simulink model "HybridFEMModel"  (Simulink 7.0)
settings: Solver=FixedStepDiscrete  SolverMode=SingleTasking  StartTime=0.0  StopTime=RunningTime  FixedStep=SampleRate  RelTol=1e-3
undefined symbols (not defined in the file): Alpham, DiscIntNeverNeededParam, Elements, gamma1, gamma2, sample, SampleRate
libraries: simulink x6
(part 2 of 4)

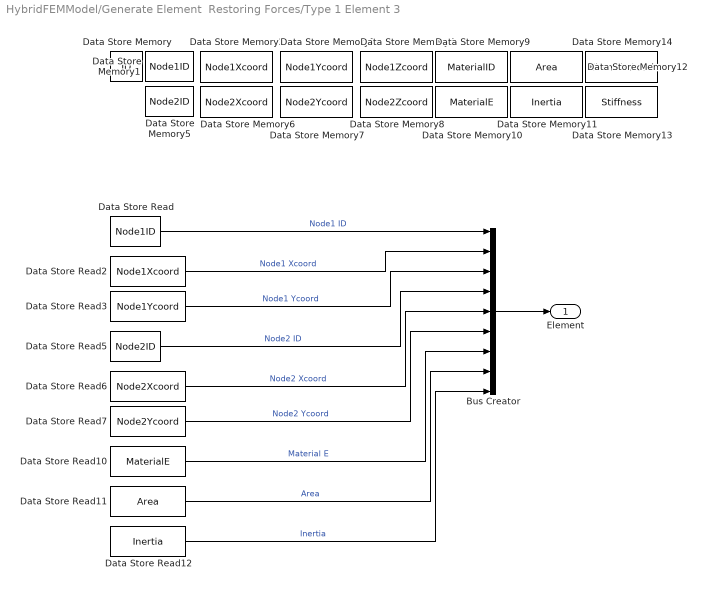
== system HybridFEMModel/Generate Element  Restoring Forces/Type 1 Element 3 ==
  Bus Creator : BusCreator  Inputs=9
  Data Store Memory : DataStoreMemory  DataStoreName=ID  InitialValue=Elements(id).ID  OutDataType=sfix(16)  OutScaling=2^0
  Data Store Memory1 : DataStoreMemory  DataStoreName=Node1ID  InitialValue=Elements(id).Nodes(1).ID  OutDataType=sfix(16)  OutScaling=2^0
  Data Store Memory10 : DataStoreMemory  DataStoreName=MaterialE  InitialValue=Elements(id).Material(1).E  OutDataType=sfix(16)  OutScaling=2^0
  Data Store Memory11 : DataStoreMemory  DataStoreName=Inertia  InitialValue=Elements(id).Inertia  OutDataType=sfix(16)  OutScaling=2^0
  Data Store Memory12 : DataStoreMemory  DataStoreName=Area  InitialValue=Elements(id).Area  OutDataType=sfix(16)  OutScaling=2^0
  Data Store Memory13 : DataStoreMemory  DataStoreName=Stiffness  InitialValue=Elements(id).Stiffness  OutDataType=sfix(16)  OutScaling=2^0
  Data Store Memory14 : DataStoreMemory  DataStoreName=ElemDistLoad  InitialValue=Elements(id).ElemDistLoad  OutDataType=sfix(16)  OutScaling=2^0
  Data Store Memory2 : DataStoreMemory  DataStoreName=Node1Xcoord  InitialValue=Elements(id).Nodes(1).Xcoord  OutDataType=sfix(16)  OutScaling=2^0
  Data Store Memory3 : DataStoreMemory  DataStoreName=Node1Ycoord  InitialValue=Elements(id).Nodes(1).Ycoord  OutDataType=sfix(16)  OutScaling=2^0
  Data Store Memory4 : DataStoreMemory  DataStoreName=Node1Zcoord  InitialValue=Elements(id).Nodes(1).Zcoord  OutDataType=sfix(16)  OutScaling=2^0
  Data Store Memory5 : DataStoreMemory  DataStoreName=Node2ID  InitialValue=Elements(id).Nodes(2).ID  OutDataType=sfix(16)  OutScaling=2^0
  Data Store Memory6 : DataStoreMemory  DataStoreName=Node2Xcoord  InitialValue=Elements(id).Nodes(2).Xcoord  OutDataType=sfix(16)  OutScaling=2^0
  Data Store Memory7 : DataStoreMemory  DataStoreName=Node2Ycoord  InitialValue=Elements(id).Nodes(2).Ycoord  OutDataType=sfix(16)  OutScaling=2^0
  Data Store Memory8 : DataStoreMemory  DataStoreName=Node2Zcoord  InitialValue=Elements(id).Nodes(2).Zcoord  OutDataType=sfix(16)  OutScaling=2^0
  Data Store Memory9 : DataStoreMemory  DataStoreName=MaterialID  InitialValue=Elements(id).Material(1).ID  OutDataType=sfix(16)  OutScaling=2^0
  Data Store Read : DataStoreRead  DataStoreName=Node1ID  SampleTime=-1
  Data Store Read10 : DataStoreRead  DataStoreName=MaterialE  SampleTime=-1
  Data Store Read11 : DataStoreRead  DataStoreName=Area  SampleTime=-1
  Data Store Read12 : DataStoreRead  DataStoreName=Inertia  SampleTime=-1
  Data Store Read2 : DataStoreRead  DataStoreName=Node1Xcoord  SampleTime=-1
  Data Store Read3 : DataStoreRead  DataStoreName=Node1Ycoord  SampleTime=-1
  Data Store Read5 : DataStoreRead  DataStoreName=Node2ID  SampleTime=-1
  Data Store Read6 : DataStoreRead  DataStoreName=Node2Xcoord  SampleTime=-1
  Data Store Read7 : DataStoreRead  DataStoreName=Node2Ycoord  SampleTime=-1
  Element : Outport  OutDataType=sfix(16)  OutScaling=2^0
  wires:
  Data Store Read12/1 -> Bus Creator/9  "Inertia"
  Data Store Read11/1 -> Bus Creator/8  "Area"
  Data Store Read10/1 -> Bus Creator/7  "Material E"
  Data Store Read7/1 -> Bus Creator/6  "Node2 Ycoord"
  Data Store Read6/1 -> Bus Creator/5  "Node2 Xcoord"
  Data Store Read5/1 -> Bus Creator/4  "Node2 ID"
  Data Store Read3/1 -> Bus Creator/3  "Node1 Ycoord"
  Data Store Read2/1 -> Bus Creator/2  "Node1 Xcoord"
  Data Store Read/1 -> Bus Creator/1  "Node1 ID"
  Bus Creator/1 -> Element/1

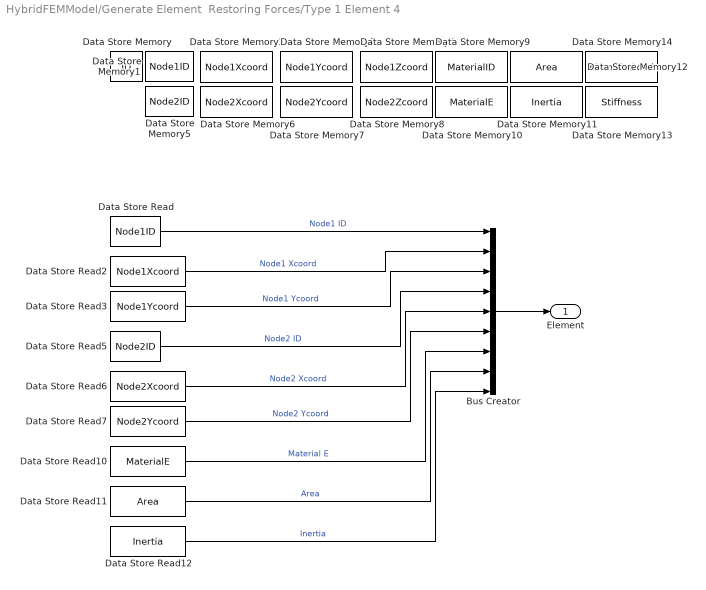
== system HybridFEMModel/Generate Element  Restoring Forces/Type 1 Element 4 ==
  Bus Creator : BusCreator  Inputs=9
  Data Store Memory : DataStoreMemory  DataStoreName=ID  InitialValue=Elements(id).ID  OutDataType=sfix(16)  OutScaling=2^0
  Data Store Memory1 : DataStoreMemory  DataStoreName=Node1ID  InitialValue=Elements(id).Nodes(1).ID  OutDataType=sfix(16)  OutScaling=2^0
  Data Store Memory10 : DataStoreMemory  DataStoreName=MaterialE  InitialValue=Elements(id).Material(1).E  OutDataType=sfix(16)  OutScaling=2^0
  Data Store Memory11 : DataStoreMemory  DataStoreName=Inertia  InitialValue=Elements(id).Inertia  OutDataType=sfix(16)  OutScaling=2^0
  Data Store Memory12 : DataStoreMemory  DataStoreName=Area  InitialValue=Elements(id).Area  OutDataType=sfix(16)  OutScaling=2^0
  Data Store Memory13 : DataStoreMemory  DataStoreName=Stiffness  InitialValue=Elements(id).Stiffness  OutDataType=sfix(16)  OutScaling=2^0
  Data Store Memory14 : DataStoreMemory  DataStoreName=ElemDistLoad  InitialValue=Elements(id).ElemDistLoad  OutDataType=sfix(16)  OutScaling=2^0
  Data Store Memory2 : DataStoreMemory  DataStoreName=Node1Xcoord  InitialValue=Elements(id).Nodes(1).Xcoord  OutDataType=sfix(16)  OutScaling=2^0
  Data Store Memory3 : DataStoreMemory  DataStoreName=Node1Ycoord  InitialValue=Elements(id).Nodes(1).Ycoord  OutDataType=sfix(16)  OutScaling=2^0
  Data Store Memory4 : DataStoreMemory  DataStoreName=Node1Zcoord  InitialValue=Elements(id).Nodes(1).Zcoord  OutDataType=sfix(16)  OutScaling=2^0
  Data Store Memory5 : DataStoreMemory  DataStoreName=Node2ID  InitialValue=Elements(id).Nodes(2).ID  OutDataType=sfix(16)  OutScaling=2^0
  Data Store Memory6 : DataStoreMemory  DataStoreName=Node2Xcoord  InitialValue=Elements(id).Nodes(2).Xcoord  OutDataType=sfix(16)  OutScaling=2^0
  Data Store Memory7 : DataStoreMemory  DataStoreName=Node2Ycoord  InitialValue=Elements(id).Nodes(2).Ycoord  OutDataType=sfix(16)  OutScaling=2^0
  Data Store Memory8 : DataStoreMemory  DataStoreName=Node2Zcoord  InitialValue=Elements(id).Nodes(2).Zcoord  OutDataType=sfix(16)  OutScaling=2^0
  Data Store Memory9 : DataStoreMemory  DataStoreName=MaterialID  InitialValue=Elements(id).Material(1).ID  OutDataType=sfix(16)  OutScaling=2^0
  Data Store Read : DataStoreRead  DataStoreName=Node1ID  SampleTime=-1
  Data Store Read10 : DataStoreRead  DataStoreName=MaterialE  SampleTime=-1
  Data Store Read11 : DataStoreRead  DataStoreName=Area  SampleTime=-1
  Data Store Read12 : DataStoreRead  DataStoreName=Inertia  SampleTime=-1
  Data Store Read2 : DataStoreRead  DataStoreName=Node1Xcoord  SampleTime=-1
  Data Store Read3 : DataStoreRead  DataStoreName=Node1Ycoord  SampleTime=-1
  Data Store Read5 : DataStoreRead  DataStoreName=Node2ID  SampleTime=-1
  Data Store Read6 : DataStoreRead  DataStoreName=Node2Xcoord  SampleTime=-1
  Data Store Read7 : DataStoreRead  DataStoreName=Node2Ycoord  SampleTime=-1
  Element : Outport  OutDataType=sfix(16)  OutScaling=2^0
  wires:
  Bus Creator/1 -> Element/1
  Data Store Read/1 -> Bus Creator/1  "Node1 ID"
  Data Store Read2/1 -> Bus Creator/2  "Node1 Xcoord"
  Data Store Read3/1 -> Bus Creator/3  "Node1 Ycoord"
  Data Store Read5/1 -> Bus Creator/4  "Node2 ID"
  Data Store Read6/1 -> Bus Creator/5  "Node2 Xcoord"
  Data Store Read7/1 -> Bus Creator/6  "Node2 Ycoord"
  Data Store Read10/1 -> Bus Creator/7  "Material E"
  Data Store Read11/1 -> Bus Creator/8  "Area"
  Data Store Read12/1 -> Bus Creator/9  "Inertia"

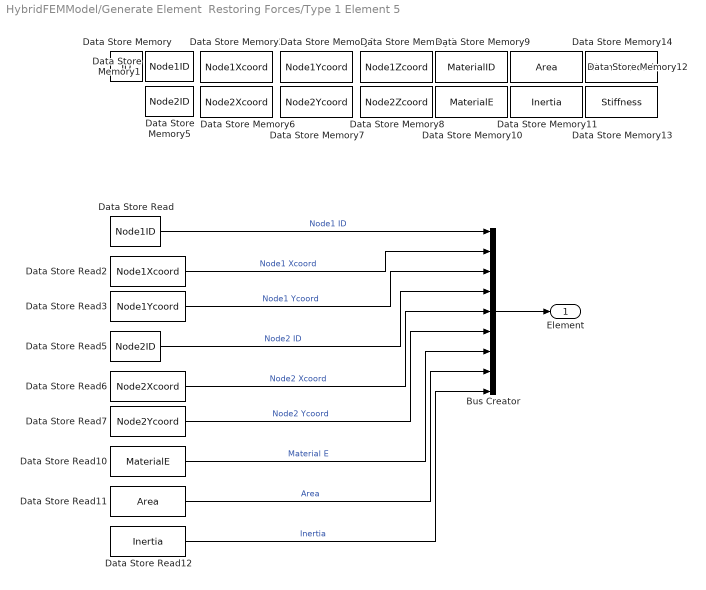
== system HybridFEMModel/Generate Element  Restoring Forces/Type 1 Element 5 ==
  Bus Creator : BusCreator  Inputs=9
  Data Store Memory : DataStoreMemory  DataStoreName=ID  InitialValue=Elements(id).ID  OutDataType=sfix(16)  OutScaling=2^0
  Data Store Memory1 : DataStoreMemory  DataStoreName=Node1ID  InitialValue=Elements(id).Nodes(1).ID  OutDataType=sfix(16)  OutScaling=2^0
  Data Store Memory10 : DataStoreMemory  DataStoreName=MaterialE  InitialValue=Elements(id).Material(1).E  OutDataType=sfix(16)  OutScaling=2^0
  Data Store Memory11 : DataStoreMemory  DataStoreName=Inertia  InitialValue=Elements(id).Inertia  OutDataType=sfix(16)  OutScaling=2^0
  Data Store Memory12 : DataStoreMemory  DataStoreName=Area  InitialValue=Elements(id).Area  OutDataType=sfix(16)  OutScaling=2^0
  Data Store Memory13 : DataStoreMemory  DataStoreName=Stiffness  InitialValue=Elements(id).Stiffness  OutDataType=sfix(16)  OutScaling=2^0
  Data Store Memory14 : DataStoreMemory  DataStoreName=ElemDistLoad  InitialValue=Elements(id).ElemDistLoad  OutDataType=sfix(16)  OutScaling=2^0
  Data Store Memory2 : DataStoreMemory  DataStoreName=Node1Xcoord  InitialValue=Elements(id).Nodes(1).Xcoord  OutDataType=sfix(16)  OutScaling=2^0
  Data Store Memory3 : DataStoreMemory  DataStoreName=Node1Ycoord  InitialValue=Elements(id).Nodes(1).Ycoord  OutDataType=sfix(16)  OutScaling=2^0
  Data Store Memory4 : DataStoreMemory  DataStoreName=Node1Zcoord  InitialValue=Elements(id).Nodes(1).Zcoord  OutDataType=sfix(16)  OutScaling=2^0
  Data Store Memory5 : DataStoreMemory  DataStoreName=Node2ID  InitialValue=Elements(id).Nodes(2).ID  OutDataType=sfix(16)  OutScaling=2^0
  Data Store Memory6 : DataStoreMemory  DataStoreName=Node2Xcoord  InitialValue=Elements(id).Nodes(2).Xcoord  OutDataType=sfix(16)  OutScaling=2^0
  Data Store Memory7 : DataStoreMemory  DataStoreName=Node2Ycoord  InitialValue=Elements(id).Nodes(2).Ycoord  OutDataType=sfix(16)  OutScaling=2^0
  Data Store Memory8 : DataStoreMemory  DataStoreName=Node2Zcoord  InitialValue=Elements(id).Nodes(2).Zcoord  OutDataType=sfix(16)  OutScaling=2^0
  Data Store Memory9 : DataStoreMemory  DataStoreName=MaterialID  InitialValue=Elements(id).Material(1).ID  OutDataType=sfix(16)  OutScaling=2^0
  Data Store Read : DataStoreRead  DataStoreName=Node1ID  SampleTime=-1
  Data Store Read10 : DataStoreRead  DataStoreName=MaterialE  SampleTime=-1
  Data Store Read11 : DataStoreRead  DataStoreName=Area  SampleTime=-1
  Data Store Read12 : DataStoreRead  DataStoreName=Inertia  SampleTime=-1
  Data Store Read2 : DataStoreRead  DataStoreName=Node1Xcoord  SampleTime=-1
  Data Store Read3 : DataStoreRead  DataStoreName=Node1Ycoord  SampleTime=-1
  Data Store Read5 : DataStoreRead  DataStoreName=Node2ID  SampleTime=-1
  Data Store Read6 : DataStoreRead  DataStoreName=Node2Xcoord  SampleTime=-1
  Data Store Read7 : DataStoreRead  DataStoreName=Node2Ycoord  SampleTime=-1
  Element : Outport  OutDataType=sfix(16)  OutScaling=2^0
  wires:
  Data Store Read12/1 -> Bus Creator/9  "Inertia"
  Data Store Read11/1 -> Bus Creator/8  "Area"
  Data Store Read10/1 -> Bus Creator/7  "Material E"
  Data Store Read7/1 -> Bus Creator/6  "Node2 Ycoord"
  Data Store Read6/1 -> Bus Creator/5  "Node2 Xcoord"
  Data Store Read5/1 -> Bus Creator/4  "Node2 ID"
  Data Store Read3/1 -> Bus Creator/3  "Node1 Ycoord"
  Data Store Read2/1 -> Bus Creator/2  "Node1 Xcoord"
  Data Store Read/1 -> Bus Creator/1  "Node1 ID"
  Bus Creator/1 -> Element/1

== system HybridFEMModel/Generate Element  Restoring Forces/Type 2 Element ==
  Bus Creator : BusCreator  Inputs=3
  Data Store Memory : DataStoreMemory  DataStoreName=ID  InitialValue=Elements(id).ID  OutDataType=sfix(16)  OutScaling=2^0
  Data Store Memory1 : DataStoreMemory  DataStoreName=Node1ID  InitialValue=Elements(id).Nodes(1).ID  OutDataType=sfix(16)  OutScaling=2^0
  Data Store Memory10 : DataStoreMemory  DataStoreName=MaterialE  InitialValue=Elements(id).Material(1).E  OutDataType=sfix(16)  OutScaling=2^0
  Data Store Memory11 : DataStoreMemory  DataStoreName=Inertia  InitialValue=Elements(id).Inertia  OutDataType=sfix(16)  OutScaling=2^0
  Data Store Memory12 : DataStoreMemory  DataStoreName=Area  InitialValue=Elements(id).Area  OutDataType=sfix(16)  OutScaling=2^0
  Data Store Memory13 : DataStoreMemory  DataStoreName=Stiffness  InitialValue=Elements(id).Stiffness  OutDataType=sfix(16)  OutScaling=2^0
  Data Store Memory14 : DataStoreMemory  DataStoreName=ElemDistLoad  InitialValue=Elements(id).ElemDistLoad  OutDataType=sfix(16)  OutScaling=2^0
  Data Store Memory2 : DataStoreMemory  DataStoreName=Node1Xcoord  InitialValue=Elements(id).Nodes(1).Xcoord  OutDataType=sfix(16)  OutScaling=2^0
  Data Store Memory3 : DataStoreMemory  DataStoreName=Node1Ycoord  InitialValue=Elements(id).Nodes(1).Ycoord  OutDataType=sfix(16)  OutScaling=2^0
  Data Store Memory4 : DataStoreMemory  DataStoreName=Node1Zcoord  InitialValue=Elements(id).Nodes(1).Zcoord  OutDataType=sfix(16)  OutScaling=2^0
  Data Store Memory5 : DataStoreMemory  DataStoreName=Node2ID  InitialValue=Elements(id).Nodes(2).ID  OutDataType=sfix(16)  OutScaling=2^0
  Data Store Memory6 : DataStoreMemory  DataStoreName=Node2Xcoord  InitialValue=Elements(id).Nodes(2).Xcoord  OutDataType=sfix(16)  OutScaling=2^0
  Data Store Memory7 : DataStoreMemory  DataStoreName=Node2Ycoord  InitialValue=Elements(id).Nodes(2).Ycoord  OutDataType=sfix(16)  OutScaling=2^0
  Data Store Memory8 : DataStoreMemory  DataStoreName=Node2Zcoord  InitialValue=Elements(id).Nodes(2).Zcoord  OutDataType=sfix(16)  OutScaling=2^0
  Data Store Memory9 : DataStoreMemory  DataStoreName=MaterialID  InitialValue=Elements(id).Material(1).ID  OutDataType=sfix(16)  OutScaling=2^0
  Data Store Read : DataStoreRead  DataStoreName=Node1ID  SampleTime=-1
  Data Store Read14 : DataStoreRead  DataStoreName=Stiffness  SampleTime=-1
  Data Store Read5 : DataStoreRead  DataStoreName=Node2ID  SampleTime=-1
  Element : Outport  OutDataType=sfix(16)  OutScaling=2^0
  wires:
  Data Store Read14/1 -> Bus Creator/3  "Stiffness"
  Data Store Read5/1 -> Bus Creator/2  "Node2 ID"
  Data Store Read/1 -> Bus Creator/1  "Node1 ID"
  Bus Creator/1 -> Element/1

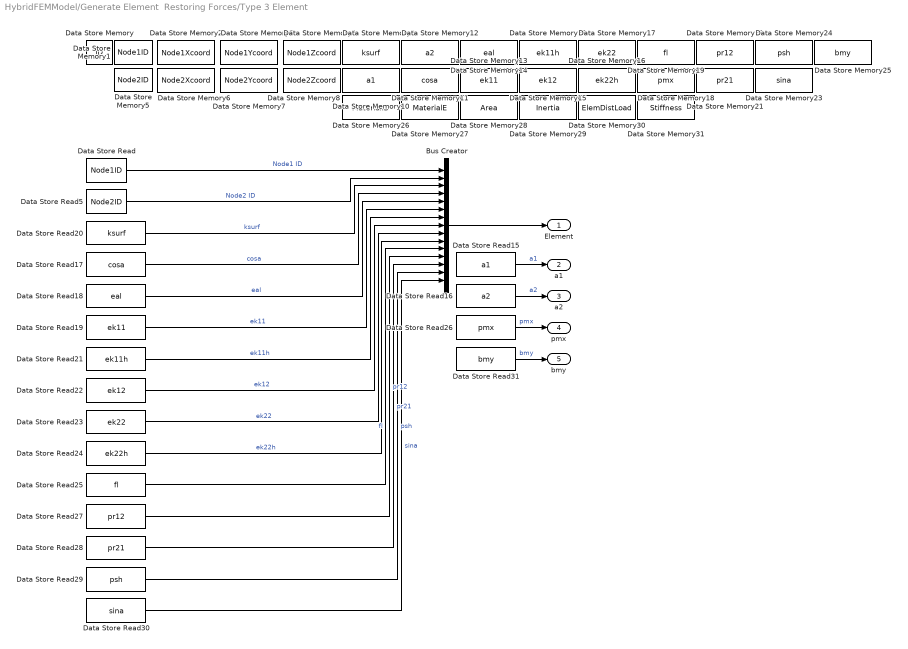
== system HybridFEMModel/Generate Element  Restoring Forces/Type 3 Element  ==
  Bus Creator : BusCreator  Inputs=15
  Data Store Memory : DataStoreMemory  DataStoreName=ID  InitialValue=Elements(id).ID  OutDataType=sfix(16)  OutScaling=2^0
  Data Store Memory1 : DataStoreMemory  DataStoreName=Node1ID  InitialValue=Elements(id).Nodes(1).ID  OutDataType=sfix(16)  OutScaling=2^0
  Data Store Memory10 : DataStoreMemory  DataStoreName=a1  InitialValue=Elements(id).a1  OutDataType=sfix(16)  OutScaling=2^0
  Data Store Memory11 : DataStoreMemory  DataStoreName=cosa  InitialValue=Elements(id).cosa  OutDataType=sfix(16)  OutScaling=2^0
  Data Store Memory12 : DataStoreMemory  DataStoreName=a2  InitialValue=Elements(id).a2  OutDataType=sfix(16)  OutScaling=2^0
  Data Store Memory13 : DataStoreMemory  DataStoreName=ek11  InitialValue=Elements(id).ek11  OutDataType=sfix(16)  OutScaling=2^0
  Data Store Memory14 : DataStoreMemory  DataStoreName=eal  InitialValue=Elements(id).eal  OutDataType=sfix(16)  OutScaling=2^0
  Data Store Memory15 : DataStoreMemory  DataStoreName=ek12  InitialValue=Elements(id).ek12  OutDataType=sfix(16)  OutScaling=2^0
  Data Store Memory16 : DataStoreMemory  DataStoreName=ek22h  InitialValue=Elements(id).ek22h  OutDataType=sfix(16)  OutScaling=2^0
  Data Store Memory17 : DataStoreMemory  DataStoreName=ek22  InitialValue=Elements(id).ek22  OutDataType=sfix(16)  OutScaling=2^0
  Data Store Memory18 : DataStoreMemory  DataStoreName=pmx  InitialValue=Elements(id).pmx  OutDataType=sfix(16)  OutScaling=2^0
  Data Store Memory19 : DataStoreMemory  DataStoreName=fl  InitialValue=Elements(id).fl  OutDataType=sfix(16)  OutScaling=2^0
  Data Store Memory2 : DataStoreMemory  DataStoreName=Node1Xcoord  InitialValue=Elements(id).Nodes(1).Xcoord  OutDataType=sfix(16)  OutScaling=2^0
  Data Store Memory20 : DataStoreMemory  DataStoreName=ek11h  InitialValue=Elements(id).ek11h  OutDataType=sfix(16)  OutScaling=2^0
  Data Store Memory21 : DataStoreMemory  DataStoreName=pr21  InitialValue=Elements(id).pr21  OutDataType=sfix(16)  OutScaling=2^0
  Data Store Memory22 : DataStoreMemory  DataStoreName=pr12  InitialValue=Elements(id).pr12  OutDataType=sfix(16)  OutScaling=2^0
  Data Store Memory23 : DataStoreMemory  DataStoreName=sina  InitialValue=Elements(id).sina  OutDataType=sfix(16)  OutScaling=2^0
  Data Store Memory24 : DataStoreMemory  DataStoreName=psh  InitialValue=Elements(id).psh  OutDataType=sfix(16)  OutScaling=2^0
  Data Store Memory25 : DataStoreMemory  DataStoreName=bmy  InitialValue=Elements(id).bmy  OutDataType=sfix(16)  OutScaling=2^0
  Data Store Memory26 : DataStoreMemory  DataStoreName=MaterialID  InitialValue=Elements(id).Material.ID  OutDataType=sfix(16)  OutScaling=2^0
  Data Store Memory27 : DataStoreMemory  DataStoreName=MaterialE  InitialValue=Elements(id).Material.E  OutDataType=sfix(16)  OutScaling=2^0
  Data Store Memory28 : DataStoreMemory  DataStoreName=Area  InitialValue=Elements(id).Area  OutDataType=sfix(16)  OutScaling=2^0
  Data Store Memory29 : DataStoreMemory  DataStoreName=Inertia  InitialValue=Elements(id).Inertia  OutDataType=sfix(16)  OutScaling=2^0
  Data Store Memory3 : DataStoreMemory  DataStoreName=Node1Ycoord  InitialValue=Elements(id).Nodes(1).Ycoord  OutDataType=sfix(16)  OutScaling=2^0
  Data Store Memory30 : DataStoreMemory  DataStoreName=ElemDistLoad  InitialValue=Elements(id).ElemDistLoad  OutDataType=sfix(16)  OutScaling=2^0
  Data Store Memory31 : DataStoreMemory  DataStoreName=Stiffness  InitialValue=Elements(id).Stiffness  OutDataType=sfix(16)  OutScaling=2^0
  Data Store Memory4 : DataStoreMemory  DataStoreName=Node1Zcoord  InitialValue=Elements(id).Nodes(1).Zcoord  OutDataType=sfix(16)  OutScaling=2^0
  Data Store Memory5 : DataStoreMemory  DataStoreName=Node2ID  InitialValue=Elements(id).Nodes(2).ID  OutDataType=sfix(16)  OutScaling=2^0
  Data Store Memory6 : DataStoreMemory  DataStoreName=Node2Xcoord  InitialValue=Elements(id).Nodes(2).Xcoord  OutDataType=sfix(16)  OutScaling=2^0
  Data Store Memory7 : DataStoreMemory  DataStoreName=Node2Ycoord  InitialValue=Elements(id).Nodes(2).Ycoord  OutDataType=sfix(16)  OutScaling=2^0
  Data Store Memory8 : DataStoreMemory  DataStoreName=Node2Zcoord  InitialValue=Elements(id).Nodes(2).Zcoord  OutDataType=sfix(16)  OutScaling=2^0
  Data Store Memory9 : DataStoreMemory  DataStoreName=ksurf  InitialValue=Elements(id).ksurf  OutDataType=sfix(16)  OutScaling=2^0
  Data Store Read : DataStoreRead  DataStoreName=Node1ID  SampleTime=-1
  Data Store Read15 : DataStoreRead  DataStoreName=a1  SampleTime=-1
  Data Store Read16 : DataStoreRead  DataStoreName=a2  SampleTime=-1
  Data Store Read17 : DataStoreRead  DataStoreName=cosa  SampleTime=-1
  Data Store Read18 : DataStoreRead  DataStoreName=eal  SampleTime=-1
  Data Store Read19 : DataStoreRead  DataStoreName=ek11  SampleTime=-1
  Data Store Read20 : DataStoreRead  DataStoreName=ksurf  SampleTime=-1
  Data Store Read21 : DataStoreRead  DataStoreName=ek11h  SampleTime=-1
  Data Store Read22 : DataStoreRead  DataStoreName=ek12  SampleTime=-1
  Data Store Read23 : DataStoreRead  DataStoreName=ek22  SampleTime=-1
  Data Store Read24 : DataStoreRead  DataStoreName=ek22h  SampleTime=-1
  Data Store Read25 : DataStoreRead  DataStoreName=fl  SampleTime=-1
  Data Store Read26 : DataStoreRead  DataStoreName=pmx  SampleTime=-1
  Data Store Read27 : DataStoreRead  DataStoreName=pr12  SampleTime=-1
  Data Store Read28 : DataStoreRead  DataStoreName=pr21  SampleTime=-1
  Data Store Read29 : DataStoreRead  DataStoreName=psh  SampleTime=-1
  Data Store Read30 : DataStoreRead  DataStoreName=sina  SampleTime=-1
  Data Store Read31 : DataStoreRead  DataStoreName=bmy  SampleTime=-1
  Data Store Read5 : DataStoreRead  DataStoreName=Node2ID  SampleTime=-1
  Element : Outport  OutDataType=sfix(16)  OutScaling=2^0
  a1 : Outport  Port=2  OutDataType=sfix(16)  OutScaling=2^0
  a2 : Outport  Port=3  OutDataType=sfix(16)  OutScaling=2^0
  pmx : Outport  Port=4  OutDataType=sfix(16)  OutScaling=2^0
  bmy : Outport  Port=5  OutDataType=sfix(16)  OutScaling=2^0
  wires:
  Bus Creator/1 -> Element/1
  Data Store Read/1 -> Bus Creator/1  "Node1 ID"
  Data Store Read5/1 -> Bus Creator/2  "Node2 ID"
  Data Store Read20/1 -> Bus Creator/3  "ksurf"
  Data Store Read17/1 -> Bus Creator/4  "cosa"
  Data Store Read18/1 -> Bus Creator/5  "eal"
  Data Store Read19/1 -> Bus Creator/6  "ek11"
  Data Store Read21/1 -> Bus Creator/7  "ek11h"
  Data Store Read22/1 -> Bus Creator/8  "ek12"
  Data Store Read23/1 -> Bus Creator/9  "ek22"
  Data Store Read24/1 -> Bus Creator/10  "ek22h"
  Data Store Read25/1 -> Bus Creator/11  "fl"
  Data Store Read27/1 -> Bus Creator/12  "pr12"
  Data Store Read28/1 -> Bus Creator/13  "pr21"
  Data Store Read29/1 -> Bus Creator/14  "psh"
  Data Store Read30/1 -> Bus Creator/15  "sina"
  Data Store Read15/1 -> a1/1  "a1"
  Data Store Read16/1 -> a2/1  "a2"
  Data Store Read26/1 -> pmx/1  "pmx"
  Data Store Read31/1 -> bmy/1  "bmy"

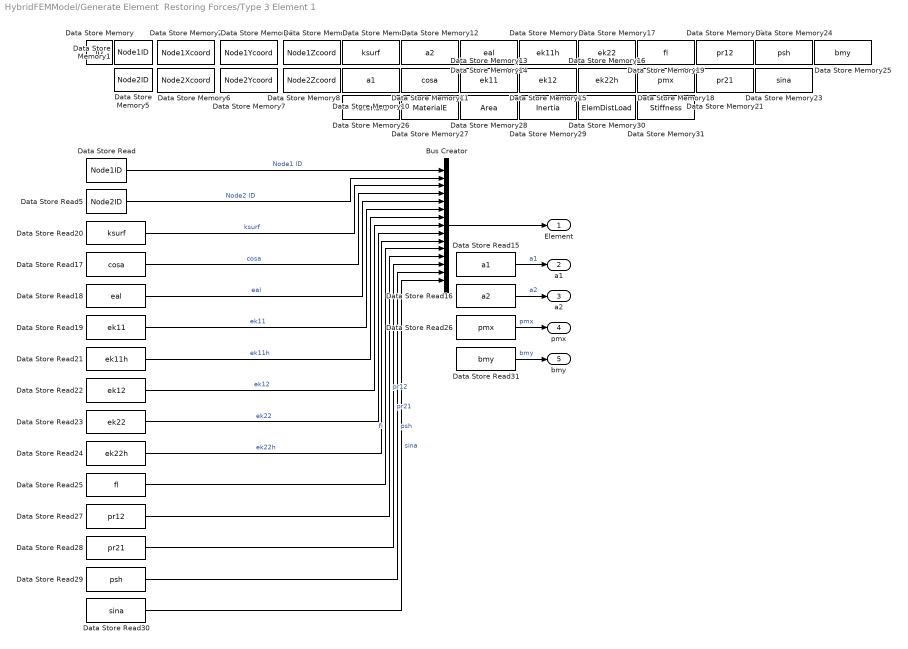
== system HybridFEMModel/Generate Element  Restoring Forces/Type 3 Element 1 ==
  Bus Creator : BusCreator  Inputs=15
  Data Store Memory : DataStoreMemory  DataStoreName=ID  InitialValue=Elements(id).ID  OutDataType=sfix(16)  OutScaling=2^0
  Data Store Memory1 : DataStoreMemory  DataStoreName=Node1ID  InitialValue=Elements(id).Nodes(1).ID  OutDataType=sfix(16)  OutScaling=2^0
  Data Store Memory10 : DataStoreMemory  DataStoreName=a1  InitialValue=Elements(id).a1  OutDataType=sfix(16)  OutScaling=2^0
  Data Store Memory11 : DataStoreMemory  DataStoreName=cosa  InitialValue=Elements(id).cosa  OutDataType=sfix(16)  OutScaling=2^0
  Data Store Memory12 : DataStoreMemory  DataStoreName=a2  InitialValue=Elements(id).a2  OutDataType=sfix(16)  OutScaling=2^0
  Data Store Memory13 : DataStoreMemory  DataStoreName=ek11  InitialValue=Elements(id).ek11  OutDataType=sfix(16)  OutScaling=2^0
  Data Store Memory14 : DataStoreMemory  DataStoreName=eal  InitialValue=Elements(id).eal  OutDataType=sfix(16)  OutScaling=2^0
  Data Store Memory15 : DataStoreMemory  DataStoreName=ek12  InitialValue=Elements(id).ek12  OutDataType=sfix(16)  OutScaling=2^0
  Data Store Memory16 : DataStoreMemory  DataStoreName=ek22h  InitialValue=Elements(id).ek22h  OutDataType=sfix(16)  OutScaling=2^0
  Data Store Memory17 : DataStoreMemory  DataStoreName=ek22  InitialValue=Elements(id).ek22  OutDataType=sfix(16)  OutScaling=2^0
  Data Store Memory18 : DataStoreMemory  DataStoreName=pmx  InitialValue=Elements(id).pmx  OutDataType=sfix(16)  OutScaling=2^0
  Data Store Memory19 : DataStoreMemory  DataStoreName=fl  InitialValue=Elements(id).fl  OutDataType=sfix(16)  OutScaling=2^0
  Data Store Memory2 : DataStoreMemory  DataStoreName=Node1Xcoord  InitialValue=Elements(id).Nodes(1).Xcoord  OutDataType=sfix(16)  OutScaling=2^0
  Data Store Memory20 : DataStoreMemory  DataStoreName=ek11h  InitialValue=Elements(id).ek11h  OutDataType=sfix(16)  OutScaling=2^0
  Data Store Memory21 : DataStoreMemory  DataStoreName=pr21  InitialValue=Elements(id).pr21  OutDataType=sfix(16)  OutScaling=2^0
  Data Store Memory22 : DataStoreMemory  DataStoreName=pr12  InitialValue=Elements(id).pr12  OutDataType=sfix(16)  OutScaling=2^0
  Data Store Memory23 : DataStoreMemory  DataStoreName=sina  InitialValue=Elements(id).sina  OutDataType=sfix(16)  OutScaling=2^0
  Data Store Memory24 : DataStoreMemory  DataStoreName=psh  InitialValue=Elements(id).psh  OutDataType=sfix(16)  OutScaling=2^0
  Data Store Memory25 : DataStoreMemory  DataStoreName=bmy  InitialValue=Elements(id).bmy  OutDataType=sfix(16)  OutScaling=2^0
  Data Store Memory26 : DataStoreMemory  DataStoreName=MaterialID  InitialValue=Elements(id).Material.ID  OutDataType=sfix(16)  OutScaling=2^0
  Data Store Memory27 : DataStoreMemory  DataStoreName=MaterialE  InitialValue=Elements(id).Material.E  OutDataType=sfix(16)  OutScaling=2^0
  Data Store Memory28 : DataStoreMemory  DataStoreName=Area  InitialValue=Elements(id).Area  OutDataType=sfix(16)  OutScaling=2^0
  Data Store Memory29 : DataStoreMemory  DataStoreName=Inertia  InitialValue=Elements(id).Inertia  OutDataType=sfix(16)  OutScaling=2^0
  Data Store Memory3 : DataStoreMemory  DataStoreName=Node1Ycoord  InitialValue=Elements(id).Nodes(1).Ycoord  OutDataType=sfix(16)  OutScaling=2^0
  Data Store Memory30 : DataStoreMemory  DataStoreName=ElemDistLoad  InitialValue=Elements(id).ElemDistLoad  OutDataType=sfix(16)  OutScaling=2^0
  Data Store Memory31 : DataStoreMemory  DataStoreName=Stiffness  InitialValue=Elements(id).Stiffness  OutDataType=sfix(16)  OutScaling=2^0
  Data Store Memory4 : DataStoreMemory  DataStoreName=Node1Zcoord  InitialValue=Elements(id).Nodes(1).Zcoord  OutDataType=sfix(16)  OutScaling=2^0
  Data Store Memory5 : DataStoreMemory  DataStoreName=Node2ID  InitialValue=Elements(id).Nodes(2).ID  OutDataType=sfix(16)  OutScaling=2^0
  Data Store Memory6 : DataStoreMemory  DataStoreName=Node2Xcoord  InitialValue=Elements(id).Nodes(2).Xcoord  OutDataType=sfix(16)  OutScaling=2^0
  Data Store Memory7 : DataStoreMemory  DataStoreName=Node2Ycoord  InitialValue=Elements(id).Nodes(2).Ycoord  OutDataType=sfix(16)  OutScaling=2^0
  Data Store Memory8 : DataStoreMemory  DataStoreName=Node2Zcoord  InitialValue=Elements(id).Nodes(2).Zcoord  OutDataType=sfix(16)  OutScaling=2^0
  Data Store Memory9 : DataStoreMemory  DataStoreName=ksurf  InitialValue=Elements(id).ksurf  OutDataType=sfix(16)  OutScaling=2^0
  Data Store Read : DataStoreRead  DataStoreName=Node1ID  SampleTime=-1
  Data Store Read15 : DataStoreRead  DataStoreName=a1  SampleTime=-1
  Data Store Read16 : DataStoreRead  DataStoreName=a2  SampleTime=-1
  Data Store Read17 : DataStoreRead  DataStoreName=cosa  SampleTime=-1
  Data Store Read18 : DataStoreRead  DataStoreName=eal  SampleTime=-1
  Data Store Read19 : DataStoreRead  DataStoreName=ek11  SampleTime=-1
  Data Store Read20 : DataStoreRead  DataStoreName=ksurf  SampleTime=-1
  Data Store Read21 : DataStoreRead  DataStoreName=ek11h  SampleTime=-1
  Data Store Read22 : DataStoreRead  DataStoreName=ek12  SampleTime=-1
  Data Store Read23 : DataStoreRead  DataStoreName=ek22  SampleTime=-1
  Data Store Read24 : DataStoreRead  DataStoreName=ek22h  SampleTime=-1
  Data Store Read25 : DataStoreRead  DataStoreName=fl  SampleTime=-1
  Data Store Read26 : DataStoreRead  DataStoreName=pmx  SampleTime=-1
  Data Store Read27 : DataStoreRead  DataStoreName=pr12  SampleTime=-1
  Data Store Read28 : DataStoreRead  DataStoreName=pr21  SampleTime=-1
  Data Store Read29 : DataStoreRead  DataStoreName=psh  SampleTime=-1
  Data Store Read30 : DataStoreRead  DataStoreName=sina  SampleTime=-1
  Data Store Read31 : DataStoreRead  DataStoreName=bmy  SampleTime=-1
  Data Store Read5 : DataStoreRead  DataStoreName=Node2ID  SampleTime=-1
  Element : Outport  OutDataType=sfix(16)  OutScaling=2^0
  a1 : Outport  Port=2  OutDataType=sfix(16)  OutScaling=2^0
  a2 : Outport  Port=3  OutDataType=sfix(16)  OutScaling=2^0
  pmx : Outport  Port=4  OutDataType=sfix(16)  OutScaling=2^0
  bmy : Outport  Port=5  OutDataType=sfix(16)  OutScaling=2^0
  wires:
  Data Store Read31/1 -> bmy/1  "bmy"
  Data Store Read26/1 -> pmx/1  "pmx"
  Data Store Read16/1 -> a2/1  "a2"
  Data Store Read15/1 -> a1/1  "a1"
  Data Store Read30/1 -> Bus Creator/15  "sina"
  Data Store Read29/1 -> Bus Creator/14  "psh"
  Data Store Read28/1 -> Bus Creator/13  "pr21"
  Data Store Read27/1 -> Bus Creator/12  "pr12"
  Data Store Read25/1 -> Bus Creator/11  "fl"
  Data Store Read24/1 -> Bus Creator/10  "ek22h"
  Data Store Read23/1 -> Bus Creator/9  "ek22"
  Data Store Read22/1 -> Bus Creator/8  "ek12"
  Data Store Read21/1 -> Bus Creator/7  "ek11h"
  Data Store Read19/1 -> Bus Creator/6  "ek11"
  Data Store Read18/1 -> Bus Creator/5  "eal"
  Data Store Read17/1 -> Bus Creator/4  "cosa"
  Data Store Read20/1 -> Bus Creator/3  "ksurf"
  Data Store Read5/1 -> Bus Creator/2  "Node2 ID"
  Data Store Read/1 -> Bus Creator/1  "Node1 ID"
  Bus Creator/1 -> Element/1

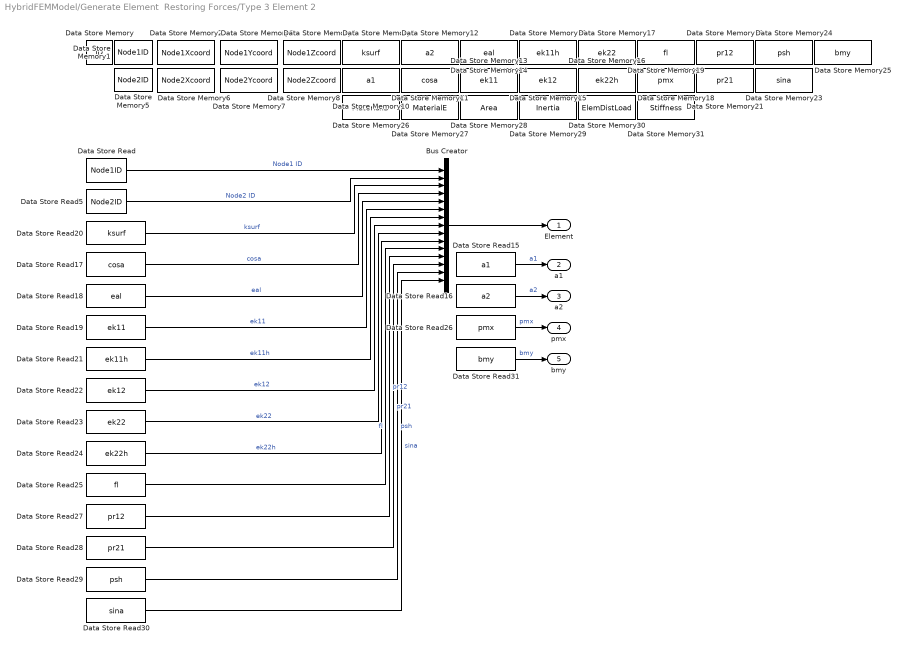
== system HybridFEMModel/Generate Element  Restoring Forces/Type 3 Element 2 ==
  Bus Creator : BusCreator  Inputs=15
  Data Store Memory : DataStoreMemory  DataStoreName=ID  InitialValue=Elements(id).ID  OutDataType=sfix(16)  OutScaling=2^0
  Data Store Memory1 : DataStoreMemory  DataStoreName=Node1ID  InitialValue=Elements(id).Nodes(1).ID  OutDataType=sfix(16)  OutScaling=2^0
  Data Store Memory10 : DataStoreMemory  DataStoreName=a1  InitialValue=Elements(id).a1  OutDataType=sfix(16)  OutScaling=2^0
  Data Store Memory11 : DataStoreMemory  DataStoreName=cosa  InitialValue=Elements(id).cosa  OutDataType=sfix(16)  OutScaling=2^0
  Data Store Memory12 : DataStoreMemory  DataStoreName=a2  InitialValue=Elements(id).a2  OutDataType=sfix(16)  OutScaling=2^0
  Data Store Memory13 : DataStoreMemory  DataStoreName=ek11  InitialValue=Elements(id).ek11  OutDataType=sfix(16)  OutScaling=2^0
  Data Store Memory14 : DataStoreMemory  DataStoreName=eal  InitialValue=Elements(id).eal  OutDataType=sfix(16)  OutScaling=2^0
  Data Store Memory15 : DataStoreMemory  DataStoreName=ek12  InitialValue=Elements(id).ek12  OutDataType=sfix(16)  OutScaling=2^0
  Data Store Memory16 : DataStoreMemory  DataStoreName=ek22h  InitialValue=Elements(id).ek22h  OutDataType=sfix(16)  OutScaling=2^0
  Data Store Memory17 : DataStoreMemory  DataStoreName=ek22  InitialValue=Elements(id).ek22  OutDataType=sfix(16)  OutScaling=2^0
  Data Store Memory18 : DataStoreMemory  DataStoreName=pmx  InitialValue=Elements(id).pmx  OutDataType=sfix(16)  OutScaling=2^0
  Data Store Memory19 : DataStoreMemory  DataStoreName=fl  InitialValue=Elements(id).fl  OutDataType=sfix(16)  OutScaling=2^0
  Data Store Memory2 : DataStoreMemory  DataStoreName=Node1Xcoord  InitialValue=Elements(id).Nodes(1).Xcoord  OutDataType=sfix(16)  OutScaling=2^0
  Data Store Memory20 : DataStoreMemory  DataStoreName=ek11h  InitialValue=Elements(id).ek11h  OutDataType=sfix(16)  OutScaling=2^0
  Data Store Memory21 : DataStoreMemory  DataStoreName=pr21  InitialValue=Elements(id).pr21  OutDataType=sfix(16)  OutScaling=2^0
  Data Store Memory22 : DataStoreMemory  DataStoreName=pr12  InitialValue=Elements(id).pr12  OutDataType=sfix(16)  OutScaling=2^0
  Data Store Memory23 : DataStoreMemory  DataStoreName=sina  InitialValue=Elements(id).sina  OutDataType=sfix(16)  OutScaling=2^0
  Data Store Memory24 : DataStoreMemory  DataStoreName=psh  InitialValue=Elements(id).psh  OutDataType=sfix(16)  OutScaling=2^0
  Data Store Memory25 : DataStoreMemory  DataStoreName=bmy  InitialValue=Elements(id).bmy  OutDataType=sfix(16)  OutScaling=2^0
  Data Store Memory26 : DataStoreMemory  DataStoreName=MaterialID  InitialValue=Elements(id).Material.ID  OutDataType=sfix(16)  OutScaling=2^0
  Data Store Memory27 : DataStoreMemory  DataStoreName=MaterialE  InitialValue=Elements(id).Material.E  OutDataType=sfix(16)  OutScaling=2^0
  Data Store Memory28 : DataStoreMemory  DataStoreName=Area  InitialValue=Elements(id).Area  OutDataType=sfix(16)  OutScaling=2^0
  Data Store Memory29 : DataStoreMemory  DataStoreName=Inertia  InitialValue=Elements(id).Inertia  OutDataType=sfix(16)  OutScaling=2^0
  Data Store Memory3 : DataStoreMemory  DataStoreName=Node1Ycoord  InitialValue=Elements(id).Nodes(1).Ycoord  OutDataType=sfix(16)  OutScaling=2^0
  Data Store Memory30 : DataStoreMemory  DataStoreName=ElemDistLoad  InitialValue=Elements(id).ElemDistLoad  OutDataType=sfix(16)  OutScaling=2^0
  Data Store Memory31 : DataStoreMemory  DataStoreName=Stiffness  InitialValue=Elements(id).Stiffness  OutDataType=sfix(16)  OutScaling=2^0
  Data Store Memory4 : DataStoreMemory  DataStoreName=Node1Zcoord  InitialValue=Elements(id).Nodes(1).Zcoord  OutDataType=sfix(16)  OutScaling=2^0
  Data Store Memory5 : DataStoreMemory  DataStoreName=Node2ID  InitialValue=Elements(id).Nodes(2).ID  OutDataType=sfix(16)  OutScaling=2^0
  Data Store Memory6 : DataStoreMemory  DataStoreName=Node2Xcoord  InitialValue=Elements(id).Nodes(2).Xcoord  OutDataType=sfix(16)  OutScaling=2^0
  Data Store Memory7 : DataStoreMemory  DataStoreName=Node2Ycoord  InitialValue=Elements(id).Nodes(2).Ycoord  OutDataType=sfix(16)  OutScaling=2^0
  Data Store Memory8 : DataStoreMemory  DataStoreName=Node2Zcoord  InitialValue=Elements(id).Nodes(2).Zcoord  OutDataType=sfix(16)  OutScaling=2^0
  Data Store Memory9 : DataStoreMemory  DataStoreName=ksurf  InitialValue=Elements(id).ksurf  OutDataType=sfix(16)  OutScaling=2^0
  Data Store Read : DataStoreRead  DataStoreName=Node1ID  SampleTime=-1
  Data Store Read15 : DataStoreRead  DataStoreName=a1  SampleTime=-1
  Data Store Read16 : DataStoreRead  DataStoreName=a2  SampleTime=-1
  Data Store Read17 : DataStoreRead  DataStoreName=cosa  SampleTime=-1
  Data Store Read18 : DataStoreRead  DataStoreName=eal  SampleTime=-1
  Data Store Read19 : DataStoreRead  DataStoreName=ek11  SampleTime=-1
  Data Store Read20 : DataStoreRead  DataStoreName=ksurf  SampleTime=-1
  Data Store Read21 : DataStoreRead  DataStoreName=ek11h  SampleTime=-1
  Data Store Read22 : DataStoreRead  DataStoreName=ek12  SampleTime=-1
  Data Store Read23 : DataStoreRead  DataStoreName=ek22  SampleTime=-1
  Data Store Read24 : DataStoreRead  DataStoreName=ek22h  SampleTime=-1
  Data Store Read25 : DataStoreRead  DataStoreName=fl  SampleTime=-1
  Data Store Read26 : DataStoreRead  DataStoreName=pmx  SampleTime=-1
  Data Store Read27 : DataStoreRead  DataStoreName=pr12  SampleTime=-1
  Data Store Read28 : DataStoreRead  DataStoreName=pr21  SampleTime=-1
  Data Store Read29 : DataStoreRead  DataStoreName=psh  SampleTime=-1
  Data Store Read30 : DataStoreRead  DataStoreName=sina  SampleTime=-1
  Data Store Read31 : DataStoreRead  DataStoreName=bmy  SampleTime=-1
  Data Store Read5 : DataStoreRead  DataStoreName=Node2ID  SampleTime=-1
  Element : Outport  OutDataType=sfix(16)  OutScaling=2^0
  a1 : Outport  Port=2  OutDataType=sfix(16)  OutScaling=2^0
  a2 : Outport  Port=3  OutDataType=sfix(16)  OutScaling=2^0
  pmx : Outport  Port=4  OutDataType=sfix(16)  OutScaling=2^0
  bmy : Outport  Port=5  OutDataType=sfix(16)  OutScaling=2^0
  wires:
  Bus Creator/1 -> Element/1
  Data Store Read/1 -> Bus Creator/1  "Node1 ID"
  Data Store Read5/1 -> Bus Creator/2  "Node2 ID"
  Data Store Read20/1 -> Bus Creator/3  "ksurf"
  Data Store Read17/1 -> Bus Creator/4  "cosa"
  Data Store Read18/1 -> Bus Creator/5  "eal"
  Data Store Read19/1 -> Bus Creator/6  "ek11"
  Data Store Read21/1 -> Bus Creator/7  "ek11h"
  Data Store Read22/1 -> Bus Creator/8  "ek12"
  Data Store Read23/1 -> Bus Creator/9  "ek22"
  Data Store Read24/1 -> Bus Creator/10  "ek22h"
  Data Store Read25/1 -> Bus Creator/11  "fl"
  Data Store Read27/1 -> Bus Creator/12  "pr12"
  Data Store Read28/1 -> Bus Creator/13  "pr21"
  Data Store Read29/1 -> Bus Creator/14  "psh"
  Data Store Read30/1 -> Bus Creator/15  "sina"
  Data Store Read15/1 -> a1/1  "a1"
  Data Store Read16/1 -> a2/1  "a2"
  Data Store Read26/1 -> pmx/1  "pmx"
  Data Store Read31/1 -> bmy/1  "bmy"

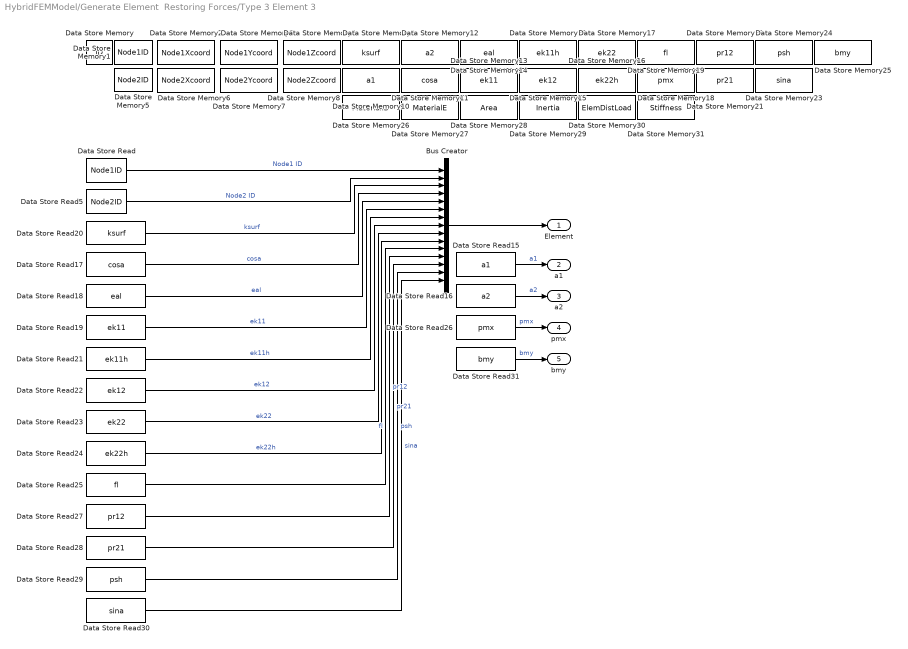
== system HybridFEMModel/Generate Element  Restoring Forces/Type 3 Element 3 ==
  Bus Creator : BusCreator  Inputs=15
  Data Store Memory : DataStoreMemory  DataStoreName=ID  InitialValue=Elements(id).ID  OutDataType=sfix(16)  OutScaling=2^0
  Data Store Memory1 : DataStoreMemory  DataStoreName=Node1ID  InitialValue=Elements(id).Nodes(1).ID  OutDataType=sfix(16)  OutScaling=2^0
  Data Store Memory10 : DataStoreMemory  DataStoreName=a1  InitialValue=Elements(id).a1  OutDataType=sfix(16)  OutScaling=2^0
  Data Store Memory11 : DataStoreMemory  DataStoreName=cosa  InitialValue=Elements(id).cosa  OutDataType=sfix(16)  OutScaling=2^0
  Data Store Memory12 : DataStoreMemory  DataStoreName=a2  InitialValue=Elements(id).a2  OutDataType=sfix(16)  OutScaling=2^0
  Data Store Memory13 : DataStoreMemory  DataStoreName=ek11  InitialValue=Elements(id).ek11  OutDataType=sfix(16)  OutScaling=2^0
  Data Store Memory14 : DataStoreMemory  DataStoreName=eal  InitialValue=Elements(id).eal  OutDataType=sfix(16)  OutScaling=2^0
  Data Store Memory15 : DataStoreMemory  DataStoreName=ek12  InitialValue=Elements(id).ek12  OutDataType=sfix(16)  OutScaling=2^0
  Data Store Memory16 : DataStoreMemory  DataStoreName=ek22h  InitialValue=Elements(id).ek22h  OutDataType=sfix(16)  OutScaling=2^0
  Data Store Memory17 : DataStoreMemory  DataStoreName=ek22  InitialValue=Elements(id).ek22  OutDataType=sfix(16)  OutScaling=2^0
  Data Store Memory18 : DataStoreMemory  DataStoreName=pmx  InitialValue=Elements(id).pmx  OutDataType=sfix(16)  OutScaling=2^0
  Data Store Memory19 : DataStoreMemory  DataStoreName=fl  InitialValue=Elements(id).fl  OutDataType=sfix(16)  OutScaling=2^0
  Data Store Memory2 : DataStoreMemory  DataStoreName=Node1Xcoord  InitialValue=Elements(id).Nodes(1).Xcoord  OutDataType=sfix(16)  OutScaling=2^0
  Data Store Memory20 : DataStoreMemory  DataStoreName=ek11h  InitialValue=Elements(id).ek11h  OutDataType=sfix(16)  OutScaling=2^0
  Data Store Memory21 : DataStoreMemory  DataStoreName=pr21  InitialValue=Elements(id).pr21  OutDataType=sfix(16)  OutScaling=2^0
  Data Store Memory22 : DataStoreMemory  DataStoreName=pr12  InitialValue=Elements(id).pr12  OutDataType=sfix(16)  OutScaling=2^0
  Data Store Memory23 : DataStoreMemory  DataStoreName=sina  InitialValue=Elements(id).sina  OutDataType=sfix(16)  OutScaling=2^0
  Data Store Memory24 : DataStoreMemory  DataStoreName=psh  InitialValue=Elements(id).psh  OutDataType=sfix(16)  OutScaling=2^0
  Data Store Memory25 : DataStoreMemory  DataStoreName=bmy  InitialValue=Elements(id).bmy  OutDataType=sfix(16)  OutScaling=2^0
  Data Store Memory26 : DataStoreMemory  DataStoreName=MaterialID  InitialValue=Elements(id).Material.ID  OutDataType=sfix(16)  OutScaling=2^0
  Data Store Memory27 : DataStoreMemory  DataStoreName=MaterialE  InitialValue=Elements(id).Material.E  OutDataType=sfix(16)  OutScaling=2^0
  Data Store Memory28 : DataStoreMemory  DataStoreName=Area  InitialValue=Elements(id).Area  OutDataType=sfix(16)  OutScaling=2^0
  Data Store Memory29 : DataStoreMemory  DataStoreName=Inertia  InitialValue=Elements(id).Inertia  OutDataType=sfix(16)  OutScaling=2^0
  Data Store Memory3 : DataStoreMemory  DataStoreName=Node1Ycoord  InitialValue=Elements(id).Nodes(1).Ycoord  OutDataType=sfix(16)  OutScaling=2^0
  Data Store Memory30 : DataStoreMemory  DataStoreName=ElemDistLoad  InitialValue=Elements(id).ElemDistLoad  OutDataType=sfix(16)  OutScaling=2^0
  Data Store Memory31 : DataStoreMemory  DataStoreName=Stiffness  InitialValue=Elements(id).Stiffness  OutDataType=sfix(16)  OutScaling=2^0
  Data Store Memory4 : DataStoreMemory  DataStoreName=Node1Zcoord  InitialValue=Elements(id).Nodes(1).Zcoord  OutDataType=sfix(16)  OutScaling=2^0
  Data Store Memory5 : DataStoreMemory  DataStoreName=Node2ID  InitialValue=Elements(id).Nodes(2).ID  OutDataType=sfix(16)  OutScaling=2^0
  Data Store Memory6 : DataStoreMemory  DataStoreName=Node2Xcoord  InitialValue=Elements(id).Nodes(2).Xcoord  OutDataType=sfix(16)  OutScaling=2^0
  Data Store Memory7 : DataStoreMemory  DataStoreName=Node2Ycoord  InitialValue=Elements(id).Nodes(2).Ycoord  OutDataType=sfix(16)  OutScaling=2^0
  Data Store Memory8 : DataStoreMemory  DataStoreName=Node2Zcoord  InitialValue=Elements(id).Nodes(2).Zcoord  OutDataType=sfix(16)  OutScaling=2^0
  Data Store Memory9 : DataStoreMemory  DataStoreName=ksurf  InitialValue=Elements(id).ksurf  OutDataType=sfix(16)  OutScaling=2^0
  Data Store Read : DataStoreRead  DataStoreName=Node1ID  SampleTime=-1
  Data Store Read15 : DataStoreRead  DataStoreName=a1  SampleTime=-1
  Data Store Read16 : DataStoreRead  DataStoreName=a2  SampleTime=-1
  Data Store Read17 : DataStoreRead  DataStoreName=cosa  SampleTime=-1
  Data Store Read18 : DataStoreRead  DataStoreName=eal  SampleTime=-1
  Data Store Read19 : DataStoreRead  DataStoreName=ek11  SampleTime=-1
  Data Store Read20 : DataStoreRead  DataStoreName=ksurf  SampleTime=-1
  Data Store Read21 : DataStoreRead  DataStoreName=ek11h  SampleTime=-1
  Data Store Read22 : DataStoreRead  DataStoreName=ek12  SampleTime=-1
  Data Store Read23 : DataStoreRead  DataStoreName=ek22  SampleTime=-1
  Data Store Read24 : DataStoreRead  DataStoreName=ek22h  SampleTime=-1
  Data Store Read25 : DataStoreRead  DataStoreName=fl  SampleTime=-1
  Data Store Read26 : DataStoreRead  DataStoreName=pmx  SampleTime=-1
  Data Store Read27 : DataStoreRead  DataStoreName=pr12  SampleTime=-1
  Data Store Read28 : DataStoreRead  DataStoreName=pr21  SampleTime=-1
  Data Store Read29 : DataStoreRead  DataStoreName=psh  SampleTime=-1
  Data Store Read30 : DataStoreRead  DataStoreName=sina  SampleTime=-1
  Data Store Read31 : DataStoreRead  DataStoreName=bmy  SampleTime=-1
  Data Store Read5 : DataStoreRead  DataStoreName=Node2ID  SampleTime=-1
  Element : Outport  OutDataType=sfix(16)  OutScaling=2^0
  a1 : Outport  Port=2  OutDataType=sfix(16)  OutScaling=2^0
  a2 : Outport  Port=3  OutDataType=sfix(16)  OutScaling=2^0
  pmx : Outport  Port=4  OutDataType=sfix(16)  OutScaling=2^0
  bmy : Outport  Port=5  OutDataType=sfix(16)  OutScaling=2^0
  wires:
  Data Store Read31/1 -> bmy/1  "bmy"
  Data Store Read26/1 -> pmx/1  "pmx"
  Data Store Read16/1 -> a2/1  "a2"
  Data Store Read15/1 -> a1/1  "a1"
  Data Store Read30/1 -> Bus Creator/15  "sina"
  Data Store Read29/1 -> Bus Creator/14  "psh"
  Data Store Read28/1 -> Bus Creator/13  "pr21"
  Data Store Read27/1 -> Bus Creator/12  "pr12"
  Data Store Read25/1 -> Bus Creator/11  "fl"
  Data Store Read24/1 -> Bus Creator/10  "ek22h"
  Data Store Read23/1 -> Bus Creator/9  "ek22"
  Data Store Read22/1 -> Bus Creator/8  "ek12"
  Data Store Read21/1 -> Bus Creator/7  "ek11h"
  Data Store Read19/1 -> Bus Creator/6  "ek11"
  Data Store Read18/1 -> Bus Creator/5  "eal"
  Data Store Read17/1 -> Bus Creator/4  "cosa"
  Data Store Read20/1 -> Bus Creator/3  "ksurf"
  Data Store Read5/1 -> Bus Creator/2  "Node2 ID"
  Data Store Read/1 -> Bus Creator/1  "Node1 ID"
  Bus Creator/1 -> Element/1

== system HybridFEMModel/Generate Element  Restoring Forces1/Generate Type 2 Element Restoring Force ==
  Displacement : Inport  OutDataType=sfix(16)  OutScaling=2^0
  Velocity : Inport  Port=2  OutDataType=sfix(16)  OutScaling=2^0
  Element : Inport  Port=3  OutDataType=sfix(16)  OutScaling=2^0
  Timestep : Inport  Port=4  OutDataType=sfix(16)  OutScaling=2^0
  Generate Actuator Command : Stateflow chart
  Act Cmd (m) : Outport  OutDataType=sfix(16)  OutScaling=2^0
  QuadRampCoeffs : Outport  Port=2  OutDataType=sfix(16)  OutScaling=2^0
  wires:
  Generate Actuator Command/1(Command) -> Act Cmd (m)/1
  Displacement/1 -> Generate Actuator Command/2(Displacement)
  Element/1 -> Generate Actuator Command/1(Element)
  Velocity/1 -> Generate Actuator Command/3(Velocity)
  Timestep/1 -> Generate Actuator Command/4(Timestep)
  Generate Actuator Command/2(QuadRampCoeffs) -> QuadRampCoeffs/1

== system HybridFEMModel/Generate Element  Restoring Forces1/Type 2 Element ==
  Bus Creator : BusCreator  Inputs=3
  Data Store Memory : DataStoreMemory  DataStoreName=ID  InitialValue=Elements(id).ID  OutDataType=sfix(16)  OutScaling=2^0
  Data Store Memory1 : DataStoreMemory  DataStoreName=Node1ID  InitialValue=Elements(id).Nodes(1).ID  OutDataType=sfix(16)  OutScaling=2^0
  Data Store Memory10 : DataStoreMemory  DataStoreName=MaterialE  InitialValue=Elements(id).Material(1).E  OutDataType=sfix(16)  OutScaling=2^0
  Data Store Memory11 : DataStoreMemory  DataStoreName=Inertia  InitialValue=Elements(id).Inertia  OutDataType=sfix(16)  OutScaling=2^0
  Data Store Memory12 : DataStoreMemory  DataStoreName=Area  InitialValue=Elements(id).Area  OutDataType=sfix(16)  OutScaling=2^0
  Data Store Memory13 : DataStoreMemory  DataStoreName=Stiffness  InitialValue=Elements(id).Stiffness  OutDataType=sfix(16)  OutScaling=2^0
  Data Store Memory14 : DataStoreMemory  DataStoreName=ElemDistLoad  InitialValue=Elements(id).ElemDistLoad  OutDataType=sfix(16)  OutScaling=2^0
  Data Store Memory2 : DataStoreMemory  DataStoreName=Node1Xcoord  InitialValue=Elements(id).Nodes(1).Xcoord  OutDataType=sfix(16)  OutScaling=2^0
  Data Store Memory3 : DataStoreMemory  DataStoreName=Node1Ycoord  InitialValue=Elements(id).Nodes(1).Ycoord  OutDataType=sfix(16)  OutScaling=2^0
  Data Store Memory4 : DataStoreMemory  DataStoreName=Node1Zcoord  InitialValue=Elements(id).Nodes(1).Zcoord  OutDataType=sfix(16)  OutScaling=2^0
  Data Store Memory5 : DataStoreMemory  DataStoreName=Node2ID  InitialValue=Elements(id).Nodes(2).ID  OutDataType=sfix(16)  OutScaling=2^0
  Data Store Memory6 : DataStoreMemory  DataStoreName=Node2Xcoord  InitialValue=Elements(id).Nodes(2).Xcoord  OutDataType=sfix(16)  OutScaling=2^0
  Data Store Memory7 : DataStoreMemory  DataStoreName=Node2Ycoord  InitialValue=Elements(id).Nodes(2).Ycoord  OutDataType=sfix(16)  OutScaling=2^0
  Data Store Memory8 : DataStoreMemory  DataStoreName=Node2Zcoord  InitialValue=Elements(id).Nodes(2).Zcoord  OutDataType=sfix(16)  OutScaling=2^0
  Data Store Memory9 : DataStoreMemory  DataStoreName=MaterialID  InitialValue=Elements(id).Material(1).ID  OutDataType=sfix(16)  OutScaling=2^0
  Data Store Read : DataStoreRead  DataStoreName=Node1ID  SampleTime=-1
  Data Store Read14 : DataStoreRead  DataStoreName=Stiffness  SampleTime=-1
  Data Store Read5 : DataStoreRead  DataStoreName=Node2ID  SampleTime=-1
  Element : Outport  OutDataType=sfix(16)  OutScaling=2^0
  wires:
  Data Store Read14/1 -> Bus Creator/3  "Stiffness"
  Data Store Read5/1 -> Bus Creator/2  "Node2 ID"
  Data Store Read/1 -> Bus Creator/1  "Node1 ID"
  Bus Creator/1 -> Element/1

== system HybridFEMModel/Linear AIC/Tracking Indicator ==
  note: TI
  note: TA
  note: A
  note: dm
  note: dc
  In1 : Inport  OutDataType=sfix(16)  OutScaling=2^0
  In2 : Inport  Port=2  OutDataType=sfix(16)  OutScaling=2^0
  A : Subsystem
  Gain : Gain  Gain=0.5  ParameterDataType=sfix(16)  ParameterScaling=2^0  OutDataType=sfix(16)  OutScaling=2^0
  Scope : Scope
      settings: SaveName=ScopeData4
  Sum : Sum  Inputs=|+-  OutDataType=sfix(16)  OutScaling=2^0
  TA : Subsystem
  Out1 : Outport  OutDataType=sfix(16)  OutScaling=2^0
  wires:
  Gain/1 -> Scope/1, Out1/1
  Sum/1 -> Gain/1
  A/1(Out1) -> Sum/1
  TA/1(Out1) -> Sum/2
  In1/1 -> TA/1(In1), A/1(In1)
  In2/1 -> TA/2(In2), A/2(In2)

== system HybridFEMModel/Linear AIC/adaptive block ==
  indicator : Inport  OutDataType=sfix(16)  OutScaling=2^0
  Discrete-Time Integrator : DiscreteIntegrator  SampleTime=sample  OutDataType=sfix(16)  OutScaling=2^0  ICPrevOutput=DiscIntNeverNeededParam  ICPrevScaledInput=DiscIntNeverNeededParam
  Gain : Gain  ParameterDataType=sfix(16)  ParameterScaling=2^0  OutDataType=sfix(16)  OutScaling=2^0
  Product : Product  OutDataType=sfix(16)  OutScaling=2^0  RndMeth=Zero
  Product1 : Product  OutDataType=sfix(16)  OutScaling=2^0  RndMeth=Zero
  Sum : Sum  Inputs=|++  OutDataType=sfix(16)  OutScaling=2^0
  gamma1 : Constant  Value=gamma1  OutDataType=sfix(16)  OutScaling=2^0
  gamma2 : Constant  Value=gamma2  OutDataType=sfix(16)  OutScaling=2^0
  Out1 : Outport  OutDataType=sfix(16)  OutScaling=2^0
  wires:
  Gain/1 -> Product1/1, Discrete-Time Integrator/1
  Product1/1 -> Sum/2
  indicator/1 -> Gain/1
  Sum/1 -> Out1/1
  Product/1 -> Sum/1
  gamma1/1 -> Product1/2
  gamma2/1 -> Product/2
  Discrete-Time Integrator/1 -> Product/1

== system HybridFEMModel/Linear AIC/inverse compensator ==
  note: dc
  note: d(alpha)
  note: dp
  In1 : Inport  OutDataType=sfix(16)  OutScaling=2^0
  In2 : Inport  Port=2  OutDataType=sfix(16)  OutScaling=2^0
  Discrete Transfer Fcn : DiscreteTransferFcn  Numerator=[1 -1]  Denominator=[1 0]  SampleTime=sample
  Product : Product  OutDataType=sfix(16)  OutScaling=2^0  RndMeth=Zero
  Scope : Scope
  Sum2 : Sum  Inputs=|++  OutDataType=sfix(16)  OutScaling=2^0
  Sum5 : Sum  Inputs=|++  OutDataType=sfix(16)  OutScaling=2^0
  Unit Delay : UnitDelay  SampleTime=sample
  alpham : Constant  Value=Alpham  OutDataType=sfix(16)  OutScaling=2^0
  Out1 : Outport  OutDataType=sfix(16)  OutScaling=2^0
  wires:
  In1/1 -> Discrete Transfer Fcn/1, Unit Delay/1
  In2/1 -> Sum5/1
  alpham/1 -> Sum5/2
  Discrete Transfer Fcn/1 -> Product/1
  Sum5/1 -> Product/2, Scope/1
  Unit Delay/1 -> Sum2/1
  Product/1 -> Sum2/2
  Sum2/1 -> Out1/1

== system HybridFEMModel/Quad Ramp Gen AIC/Tracking Indicator ==
  note: dc
  note: dm
  note: A
  note: TA
  note: TI
  In1 : Inport  OutDataType=sfix(16)  OutScaling=2^0
  In2 : Inport  Port=2  OutDataType=sfix(16)  OutScaling=2^0
  A : Subsystem
  Gain : Gain  Gain=0.5  ParameterDataType=sfix(16)  ParameterScaling=2^0  OutDataType=sfix(16)  OutScaling=2^0
  Scope : Scope
      settings: SaveName=ScopeData4
  Sum : Sum  Inputs=|+-  OutDataType=sfix(16)  OutScaling=2^0
  TA : Subsystem
  Out1 : Outport  OutDataType=sfix(16)  OutScaling=2^0
  wires:
  In2/1 -> A/2(In2), TA/2(In2)
  In1/1 -> A/1(In1), TA/1(In1)
  TA/1(Out1) -> Sum/2
  A/1(Out1) -> Sum/1
  Sum/1 -> Gain/1
  Gain/1 -> Out1/1, Scope/1

== system HybridFEMModel/Quad Ramp Gen AIC/adaptive block ==
  indicator : Inport  OutDataType=sfix(16)  OutScaling=2^0
  Discrete-Time Integrator : DiscreteIntegrator  SampleTime=sample  OutDataType=sfix(16)  OutScaling=2^0  ICPrevOutput=DiscIntNeverNeededParam  ICPrevScaledInput=DiscIntNeverNeededParam
  Gain : Gain  ParameterDataType=sfix(16)  ParameterScaling=2^0  OutDataType=sfix(16)  OutScaling=2^0
  Product : Product  OutDataType=sfix(16)  OutScaling=2^0  RndMeth=Zero
  Product1 : Product  OutDataType=sfix(16)  OutScaling=2^0  RndMeth=Zero
  Sum : Sum  Inputs=|++  OutDataType=sfix(16)  OutScaling=2^0
  gamma1 : Constant  Value=gamma1  OutDataType=sfix(16)  OutScaling=2^0
  gamma2 : Constant  Value=gamma2  OutDataType=sfix(16)  OutScaling=2^0
  Out1 : Outport  OutDataType=sfix(16)  OutScaling=2^0
  wires:
  Discrete-Time Integrator/1 -> Product/1
  gamma2/1 -> Product/2
  gamma1/1 -> Product1/2
  Product/1 -> Sum/1
  Sum/1 -> Out1/1
  indicator/1 -> Gain/1
  Product1/1 -> Sum/2
  Gain/1 -> Discrete-Time Integrator/1, Product1/1
